simulink model "Nonlinear_Observer_v3"  (R2021a)
settings: Solver=VariableStepAuto  StartTime=0.0  StopTime=20  RelTol=1e-3
settings Model: Creator=JianFongLee  LastModifiedBy=JianFongLee

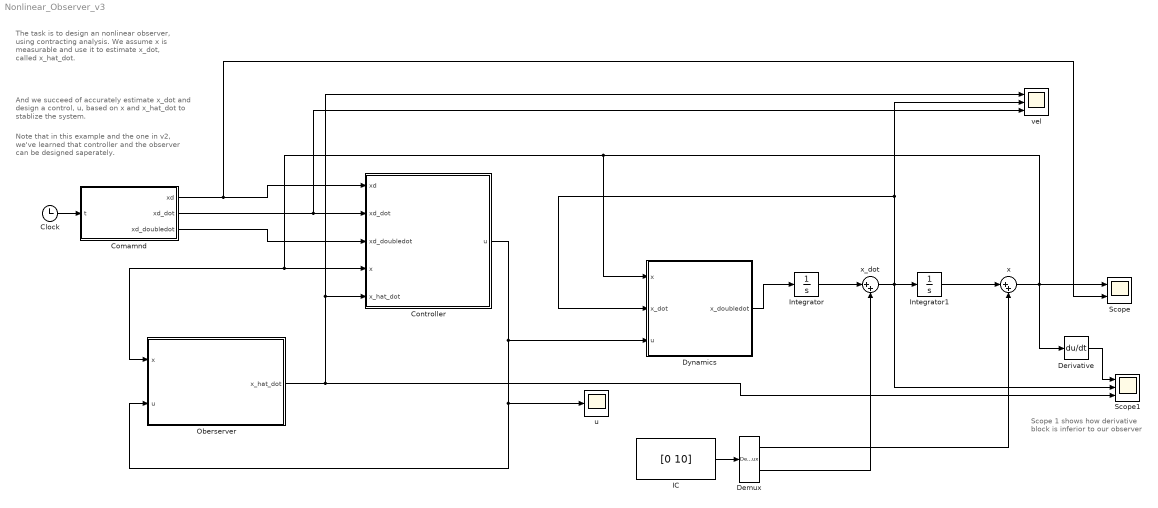
== system Nonlinear_Observer_v3 ==
  note: Scope 1 shows how derivative
      | block is inferior to our observer
  note: Note that in this example and the one in v2,
      | we've learned that controller and the observer
      | can be designed saperately.
  note: And we succeed of accurately estimate x_dot
      | and design a control, u, based on x and x_hat_dot
      | to stablize the system.
  note: The task is to design an nonlinear observer,
      | using contracting analysis.
      | We assume x is measurable and use it to
      | estimate x_dot, called x_hat_dot.
  Clock : Clock
  Comamnd : MATLAB Function  TreatAsAtomicUnit=on
  Controller : MATLAB Function  TreatAsAtomicUnit=on
  Demux : Demux  Outputs=2
      settings: DisplayOption=none
  Derivative : Derivative
  Dynamics : MATLAB Function  TreatAsAtomicUnit=on
  IC : Constant  Value=[0 10]
  Integrator : Integrator
  Integrator1 : Integrator
  Oberserver : Subsystem
  Scope : Scope  NumInputPorts=2
  Scope1 : Scope  NumInputPorts=3
  u : Scope
  vel : Scope  NumInputPorts=3
  x : Sum  Inputs=|++
  x_dot : Sum  Inputs=|++
  wires:
  IC/1 -> Demux/1
  Dynamics/1(x_doubledot) -> Integrator/1
  Integrator/1 -> x_dot/1
  Demux/2 -> x_dot/2
  x_dot/1 -> vel/2, Dynamics/2(x_dot), Scope1/2, Integrator1/1
  Integrator1/1 -> x/1
  Demux/1 -> x/2
  x/1 -> Derivative/1, Controller/4(x), Oberserver/1(x), Dynamics/1(x), Scope/1
  Clock/1 -> Comamnd/1(t)
  Comamnd/2(xd_dot) -> vel/3, Controller/2(xd_dot)
  Comamnd/3(xd_doubledot) -> Controller/3(xd_doubledot)
  Oberserver/1(x_hat_dot) -> Scope1/3, vel/1, Controller/5(x_hat_dot)
  Controller/1(u) -> Dynamics/3(u), u/1, Oberserver/2(u)
  Comamnd/1(xd) -> Scope/2, Controller/1(xd)
  Derivative/1 -> Scope1/1

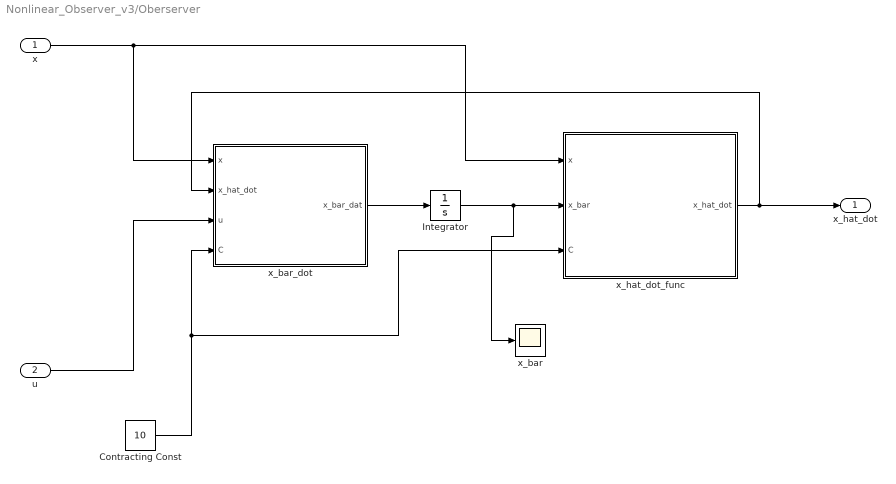
== system Nonlinear_Observer_v3/Oberserver ==
  x : Inport
  u : Inport  Port=2
  Contracting Const : Constant  Value=10
  Integrator : Integrator
  x_bar : Scope
  x_bar_dot : MATLAB Function  TreatAsAtomicUnit=on
  x_hat_dot_func : MATLAB Function  TreatAsAtomicUnit=on
  x_hat_dot : Outport
  wires:
  x/1 -> x_bar_dot/1(x), x_hat_dot_func/1(x)
  u/1 -> x_bar_dot/3(u)
  x_bar_dot/1(x_bar_dat) -> Integrator/1
  Integrator/1 -> x_bar/1, x_hat_dot_func/2(x_bar)
  x_hat_dot_func/1(x_hat_dot) -> x_hat_dot/1, x_bar_dot/2(x_hat_dot)
  Contracting Const/1 -> x_hat_dot_func/3(C), x_bar_dot/4(C)

== matlab function Nonlinear_Observer_v3/Controller ==
  data: xd input; xd_dot input; xd_doubledot input; x input; u output; x_hat_dot input
function u = fcn(xd,xd_dot,xd_doubledot,x,x_hat_dot)
%%% Controller here
%%% Note that x_dot is not measureable,
%%% so we build an obersver for x_dot,called x_hat_dot
lemmda = 1.2;
R = 10;     %%%Restrain of u
k1 = 0.2;
x_telda = xd- x;
x_teldadot = xd_dot - x_hat_dot;
s = x_teldadot + lemmda*x_telda;
u = xd_doubledot + 0.05*x^3 - 0.15*(x^2)*x_hat_dot + x*x_hat_dot...
    - 0.6*x + lemmda*x_teldadot + x_telda - k1*s;

% if(u>R)
%     u = R;
% elseif(u<-R)
%     u = -R;
% end
end

== matlab function Nonlinear_Observer_v3/Dynamics ==
  data: x input; x_dot input; u input; x_doubledot output
function x_doubledot = fcn(x,x_dot,u)
%%% The dynamics of the system
%%% Note that the dynamics is somewhat tricky here
%%% It can't have dynamic parts which can't be calculted by x,
%%% like (x_dot)^2
x_doubledot = -0.05*(x^3) + 0.15*(x^2)*x_dot - x*x_dot + 0.6*x + u;
end

== matlab function Nonlinear_Observer_v3/Oberserver/x_bar_dot ==
  data: x input; x_hat_dot input; u input; x_bar_dat output; C input
function x_bar_dat = fcn(x,x_hat_dot,u,C)

   
x_bar_dat = -0.05*x^3 + 0.6*x + u - C*x_hat_dot;
        
end

== matlab function Nonlinear_Observer_v3/Oberserver/x_hat_dot_func ==
  data: x input; x_bar input; x_hat_dot output; C input
function x_hat_dot = fcn(x,x_bar,C)
%%%
x_hat_dot = x_bar + C*x - 0.5*x^2 + 0.15/3*(x^3);
end

== matlab function Nonlinear_Observer_v3/Comamnd ==
  data: t input; xd output; xd_dot output; xd_doubledot output
function [xd,xd_dot,xd_doubledot]= fcn(t)
%%% Tracking states

%%% sinusoidal signal, rather good
A = 2;
w = 1.5;
xd = A*sin(w*t);
xd_dot = A*w*cos(w*t);
xd_doubledot = -A*(w^2)*sin(w*t);

%%% polynomial signal, rather poor, esp for higher order terms
% xd = 0.01*t^3 - 0.8*t + 2;
% xd_dot = 0.03*t^2 - 0.8;
% xd_doubledot = 0.06;
end
